simulink model "planar_kinctrl2"  (R2020b)
settings: Solver=VariableStepAuto  StartTime=0.0  StopTime=10.0  RelTol=1e-3
values from neighbouring files (symbols this model uses):
  q0 = [pi -pi/2 -pi/2]    [planar_mdl.m]
libraries: roblocks x3
settings Model: Creator=lucas  LastModifiedBy=lucas

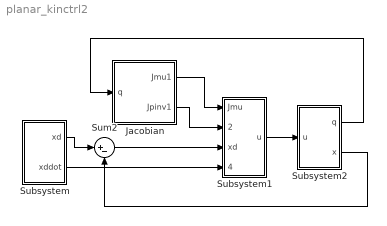
== system planar_kinctrl2 ==
  Jacobian : Subsystem
  Subsystem : Subsystem
  Subsystem1 : Subsystem
  Subsystem2 : Subsystem
  Sum2 : Sum  Inputs=|+-
  wires:
  Subsystem/1(xd) -> Sum2/1
  Jacobian/1(Jmu1) -> Subsystem1/1(Jmu)
  Jacobian/2(Jpinv1) -> Subsystem1/2(Jpinv)
  Sum2/1 -> Subsystem1/3(xd)
  Subsystem/2(xddot) -> Subsystem1/4(xddot)
  Subsystem1/1(u) -> Subsystem2/1(u)
  Subsystem2/1(q) -> Jacobian/1(q)
  Subsystem2/2(x) -> Sum2/2

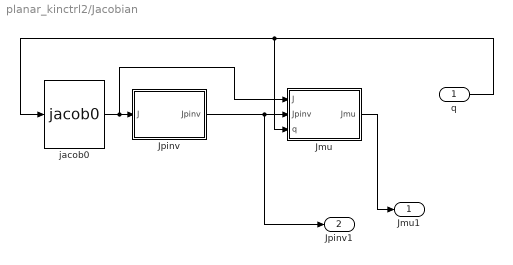
== system planar_kinctrl2/Jacobian ==
  q : Inport
  Jmu : MATLAB Function  TreatAsAtomicUnit=on
  Jpinv : MATLAB Function  TreatAsAtomicUnit=on
  "jacob0 " : roblocks/Arm/jacob0   robot=planar
  Jmu1 : Outport
  Jpinv1 : Outport  Port=2
  wires:
  "jacob0 "/1 -> Jmu/1(J), Jpinv/1(J)
  Jmu/1(Jmu) -> Jmu1/1
  q/1 -> Jmu/3(q), "jacob0 "/1
  Jpinv/1(Jpinv) -> Jpinv1/1, Jmu/2(Jpinv)

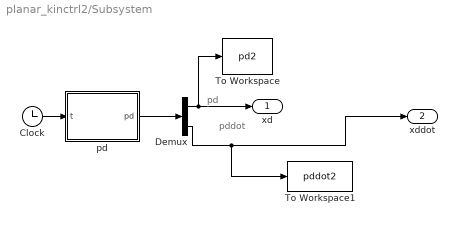
== system planar_kinctrl2/Subsystem ==
  note: pd
  note: pddot
  Clock : Clock
  Demux : Demux  Outputs=2
  To Workspace : ToWorkspace  VariableName=pd2  SaveFormat=Timeseries  SampleTime=-1
  To Workspace1 : ToWorkspace  VariableName=pddot2  SaveFormat=Timeseries  SampleTime=-1
  pd : MATLAB Function  TreatAsAtomicUnit=on
  xd : Outport
  xddot : Outport  Port=2
  wires:
  Demux/2 -> xddot/1, To Workspace1/1
  Demux/1 -> xd/1, To Workspace/1
  Clock/1 -> pd/1(t)
  pd/1(pd) -> Demux/1

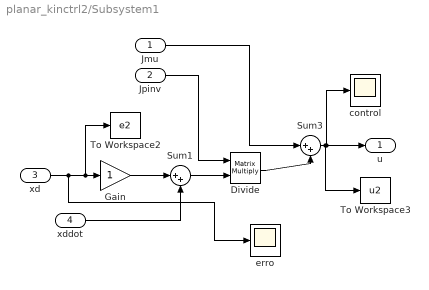
== system planar_kinctrl2/Subsystem1 ==
  Jmu : Inport
  Jpinv : Inport  Port=2
  xd : Inport  Port=3
  xddot : Inport  Port=4
  Divide : Product  Inputs=**  Multiplication=Matrix(*)
  Gain : Gain
  Sum1 : Sum  Inputs=|++
  Sum3 : Sum  Inputs=|++
  To Workspace2 : ToWorkspace  VariableName=e2  SaveFormat=Timeseries  SampleTime=-1
  To Workspace3 : ToWorkspace  VariableName=u2  SaveFormat=Timeseries  SampleTime=-1
  control : Scope
  erro : Scope
  u : Outport
  wires:
  Sum3/1 -> To Workspace3/1, u/1, control/1
  Jmu/1 -> Sum3/1
  xd/1 -> erro/1, To Workspace2/1, Gain/1
  Divide/1 -> Sum3/2
  Sum1/1 -> Divide/2
  Jpinv/1 -> Divide/1
  Gain/1 -> Sum1/1
  xddot/1 -> Sum1/2

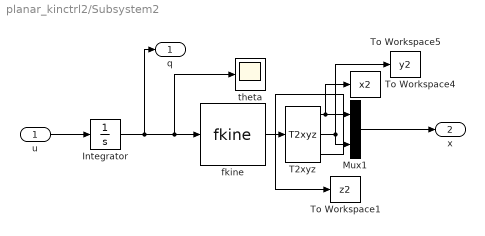
== system planar_kinctrl2/Subsystem2 ==
  u : Inport
  Integrator : Integrator  InitialCondition=q0
  Mux1 : Mux  Inputs=2
  T2xyz : roblocks/Toolbox/T2xyz
  To Workspace1 : ToWorkspace  VariableName=z2  SaveFormat=Timeseries  SampleTime=-1
  To Workspace4 : ToWorkspace  VariableName=x2  SaveFormat=Timeseries  SampleTime=-1
  To Workspace5 : ToWorkspace  VariableName=y2  SaveFormat=Timeseries  SampleTime=-1
  fkine : roblocks/Arm/fkine  robot=planar
  theta : Scope
  q : Outport
  x : Outport  Port=2
  wires:
  Integrator/1 -> q/1, theta/1, fkine/1
  Mux1/1 -> x/1
  fkine/1 -> T2xyz/1
  T2xyz/2 -> To Workspace5/1, Mux1/2
  T2xyz/1 -> To Workspace4/1, Mux1/1
  u/1 -> Integrator/1
  T2xyz/3 -> To Workspace1/1

== matlab function planar_kinctrl2/Subsystem/pd ==
  data: t input; pd output
function pd  = fcn(t)

xd = [0.25*(1-cos(pi*t)) 0.25*(2+sin(pi*t))]';
xddot = [0.25*pi*sin(pi*t) 0.25*pi*cos(pi*t)]';

pd=[xd;xddot];

== matlab function planar_kinctrl2/Jacobian/Jpinv ==
  data: J input; Jpinv output
function Jpinv = Jpinv(J)
    J = J(1:2,1:3);
    Jpinv = pinv(J);

== matlab function planar_kinctrl2/Jacobian/Jmu ==
  data: J input; Jmu output; Jpinv input; q input
function Jmu = fcn(J,Jpinv,q)
    K0 = 1;
    mu = (-K0/(3*pi^2))*[q(1)/16 q(2) q(3)+pi]';
    J = J(1:2,1:3);
    J = (eye(3,3) - Jpinv*J);
    Jmu = J*mu;
